simulink model "distrubance_Tracking_Integral_for_first_desired_poles"  (R2021b)
settings: Solver=VariableStepAuto  StartTime=0.0  StopTime=20  RelTol=1e-3
undefined symbols (not defined in the file): A, B, C, KI1_1, KI1_2
settings Model: Creator=nima8  LastModifiedBy=nima8

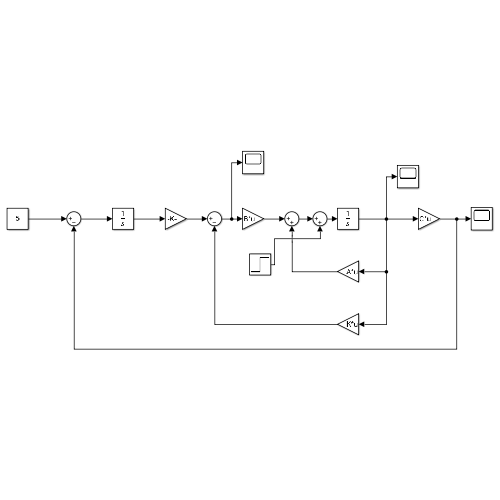
[thumbnail: Simulink's stored preview of the top-level diagram]
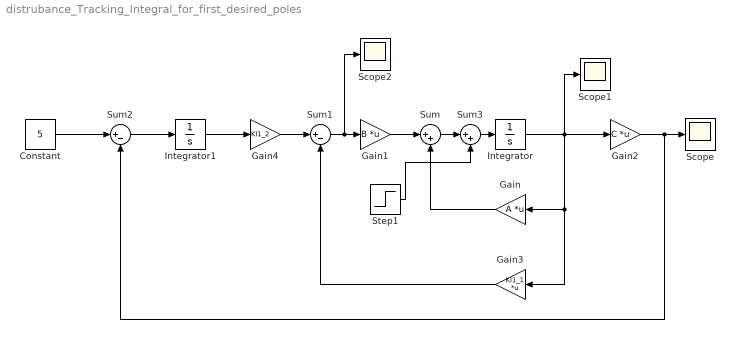
== system distrubance_Tracking_Integral_for_first_desired_poles ==
  Constant : Constant  Value=5
  Gain : Gain  Gain=A  Multiplication=Matrix(K*u)
  Gain1 : Gain  Gain=B  Multiplication=Matrix(K*u)
  Gain2 : Gain  Gain=C  Multiplication=Matrix(K*u)
  Gain3 : Gain  Gain=KI1_1  Multiplication=Matrix(K*u)
  Gain4 : Gain  Gain=KI1_2
  Integrator : Integrator  InitialCondition=[1 0.5 -1 2]
  Integrator1 : Integrator  InitialCondition=2
  Scope : Scope
  Scope1 : Scope
  Scope2 : Scope
  Step1 : Step  Time=10  SampleTime=0
  Sum : Sum  Inputs=|++
  Sum1 : Sum  Inputs=|+-
  Sum2 : Sum  Inputs=|+-
  Sum3 : Sum  Inputs=|++
  wires:
  Gain2/1 -> Sum2/2, Scope/1
  Constant/1 -> Sum2/1
  Integrator1/1 -> Gain4/1
  Sum2/1 -> Integrator1/1
  Gain4/1 -> Sum1/1
  Gain1/1 -> Sum/1
  Gain3/1 -> Sum1/2
  Integrator/1 -> Scope1/1, Gain/1, Gain3/1, Gain2/1
  Gain/1 -> Sum/2
  Sum/1 -> Sum3/1
  Sum3/1 -> Integrator/1
  Step1/1 -> Sum3/2
  Sum1/1 -> Scope2/1, Gain1/1
